simulink model "Adaptive_control"  (R2018a)
settings: Solver=ode45  StartTime=0.0  StopTime=20  RelTol=1e-3
libraries: simulink x3
settings Model: Creator=Chi  LastModifiedBy=Chi

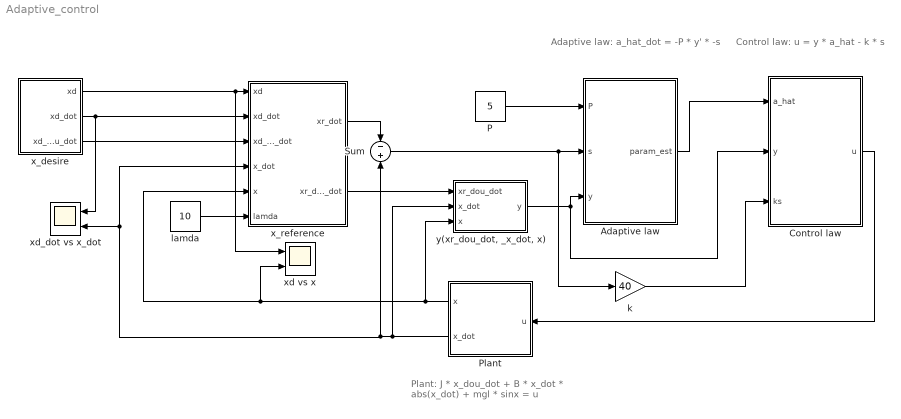
== system Adaptive_control ==
  note: Adaptive law:
      | a_hat_dot = -P * y' * -s
  note: Control law:
      | u = y * a_hat - k * s
  note: Plant:
      | J * x_dou_dot + B * x_dot * abs(x_dot) + mgl * sinx = u
  Adaptive law : Subsystem
  Control law : Subsystem
  P : Constant  Value=5
  Plant : Subsystem
  Sum : Sum  Inputs=-|+
  k : Gain  Gain=40
  lamda : Constant  Value=10
  x_desire : Subsystem
  x_reference : Subsystem
  xd vs x : Scope  NumInputPorts=2
  xd_dot vs x_dot : Scope  NumInputPorts=2
  "y(xr_dou_dot, _x_dot, x)" : MATLAB Function  TreatAsAtomicUnit=on
  wires:
  x_desire/1(xd) -> xd vs x/1, x_reference/1("xd ")
  x_desire/2("xd_dot ") -> xd_dot vs x_dot/1, x_reference/2(xd_dot)
  x_desire/3(xd_dou_dot) -> x_reference/3(xd_dou_dot)
  Plant/2(x_dot) -> "y(xr_dou_dot, _x_dot, x)"/2(x_dot), Sum/2, xd_dot vs x_dot/2, x_reference/4(x_dot)
  Plant/1(x) -> "y(xr_dou_dot, _x_dot, x)"/3(x), xd vs x/2, x_reference/5(x)
  x_reference/1(xr_dot) -> Sum/1
  lamda/1 -> x_reference/6(lamda)
  x_reference/2(xr_dou_dot) -> "y(xr_dou_dot, _x_dot, x)"/1(xr_dou_dot)
  P/1 -> Adaptive law/1(P)
  Sum/1 -> k/1, Adaptive law/2(s)
  "y(xr_dou_dot, _x_dot, x)"/1(y) -> Adaptive law/3(y), Control law/2(y)
  Adaptive law/1(param_est) -> Control law/1(a_hat)
  k/1 -> Control law/3(ks)
  Control law/1(u) -> Plant/1(u)

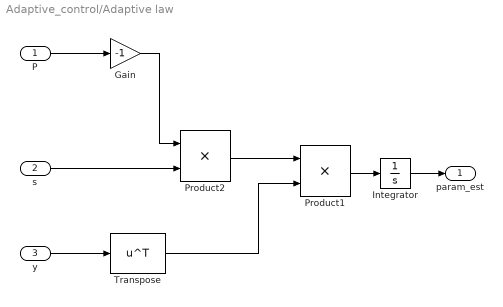
== system Adaptive_control/Adaptive law ==
  P : Inport
  s : Inport  Port=2
  y : Inport  Port=3
  Gain : Gain  Gain=-1
  Integrator : Integrator
  Product1 : Product  RndMeth=Zero
  Product2 : Product  RndMeth=Zero
  Transpose : Math  Operator=transpose  SaturateOnIntegerOverflow=on
  param_est : Outport
  wires:
  Integrator/1 -> param_est/1
  P/1 -> Gain/1
  y/1 -> Transpose/1
  Transpose/1 -> Product1/2
  s/1 -> Product2/2
  Product2/1 -> Product1/1
  Product1/1 -> Integrator/1
  Gain/1 -> Product2/1

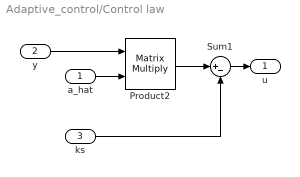
== system Adaptive_control/Control law ==
  a_hat : Inport
  y : Inport  Port=2
  ks : Inport  Port=3
  Product2 : Product  Multiplication=Matrix(*)  RndMeth=Zero
  Sum1 : Sum  Inputs=|+-
  u : Outport
  wires:
  Product2/1 -> Sum1/1
  ks/1 -> Sum1/2
  Sum1/1 -> u/1
  a_hat/1 -> Product2/2
  y/1 -> Product2/1

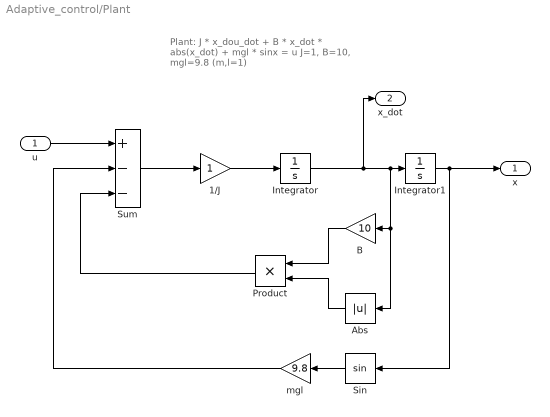
== system Adaptive_control/Plant ==
  note: Plant:
      | J * x_dou_dot + B * x_dot * abs(x_dot) + mgl * sinx = u
      | J=1, B=10, mgl=9.8 (m,l=1)
  u : Inport
  1/J : Gain
  Abs : Abs
  B : Gain  Gain=10
  Integrator : Integrator
  Integrator1 : Integrator
  Product : Product
  Sin : Trigonometry
  Sum : Sum  Inputs=+--
  mgl : Gain  Gain=9.8
  x : Outport
  x_dot : Outport  Port=2
  wires:
  Integrator/1 -> x_dot/1, Abs/1, B/1, Integrator1/1
  Product/1 -> Sum/3
  Sin/1 -> mgl/1
  1/J/1 -> Integrator/1
  Sum/1 -> 1/J/1
  mgl/1 -> Sum/2
  Integrator1/1 -> x/1, Sin/1
  u/1 -> Sum/1
  B/1 -> Product/1
  Abs/1 -> Product/2

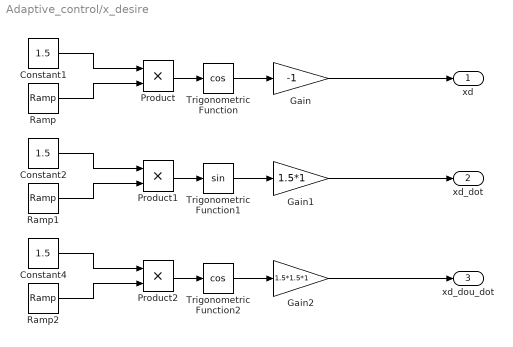
== system Adaptive_control/x_desire ==
  Constant1 : Constant  Value=1.5
  Constant2 : Constant  Value=1.5
  Constant4 : Constant  Value=1.5
  Gain : Gain  Gain=-1
  Gain1 : Gain  Gain=1.5*1
  Gain2 : Gain  Gain=1.5*1.5*1
  Product : Product  RndMeth=Zero
  Product1 : Product  RndMeth=Zero
  Product2 : Product  RndMeth=Zero
  Ramp : simulink/Sources/Ramp  slope=1  start=0  InitialOutput=0
  Ramp1 : simulink/Sources/Ramp  slope=1  start=0  InitialOutput=0
  Ramp2 : simulink/Sources/Ramp  slope=1  start=0  InitialOutput=0
  Trigonometric Function : Trigonometry  Operator=cos
  Trigonometric Function1 : Trigonometry
  Trigonometric Function2 : Trigonometry  Operator=cos
  xd : Outport
  "xd_dot " : Outport  Port=2
  xd_dou_dot : Outport  Port=3
  wires:
  Ramp2/1 -> Product2/2
  Ramp1/1 -> Product1/2
  Constant2/1 -> Product1/1
  Gain2/1 -> xd_dou_dot/1
  Constant4/1 -> Product2/1
  Trigonometric Function1/1 -> Gain1/1
  Trigonometric Function2/1 -> Gain2/1
  Product1/1 -> Trigonometric Function1/1
  Gain1/1 -> "xd_dot "/1
  Constant1/1 -> Product/1
  Trigonometric Function/1 -> Gain/1
  Product/1 -> Trigonometric Function/1
  Product2/1 -> Trigonometric Function2/1
  Ramp/1 -> Product/2
  Gain/1 -> xd/1

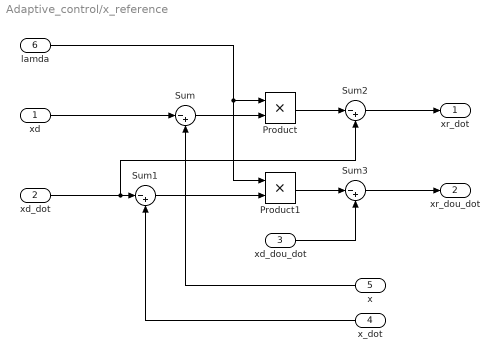
== system Adaptive_control/x_reference ==
  "xd " : Inport
  xd_dot : Inport  Port=2
  xd_dou_dot : Inport  Port=3
  x_dot : Inport  Port=4
  x : Inport  Port=5
  lamda : Inport  Port=6
  Product : Product
  Product1 : Product
  Sum{,1..3} (4 alike) : Sum  Inputs=|-+
  xr_dot : Outport
  xr_dou_dot : Outport  Port=2
  wires:
  Sum3/1 -> xr_dou_dot/1
  lamda/1 -> Product1/1, Product/1
  Product1/1 -> Sum3/1
  Sum1/1 -> Product1/2
  xd_dot/1 -> Sum2/2, Sum1/1
  Sum/1 -> Product/2
  Product/1 -> Sum2/1
  Sum2/1 -> xr_dot/1
  "xd "/1 -> Sum/1
  xd_dou_dot/1 -> Sum3/2
  x_dot/1 -> Sum1/2
  x/1 -> Sum/2

== matlab function Adaptive_control/y(xr_dou_dot, _x_dot, x) ==
  data: xr_dou_dot input; y output; x_dot input; x input
function y = fcn(xr_dou_dot, x_dot, x)

y = [xr_dou_dot, x_dot*abs(x_dot), sin(x)];

end
